simulink model "TST_InjCrv_PoI2AddCor"  (R2016b)
settings: Solver=FixedStepDiscrete  StartTime=0.0  StopTime=simTime  FixedStep=sampleTime  RelTol=1e-3
values from neighbouring files (symbols this model uses):
  testCase = 1    [initTST_InjCrv_PoI2AddCor_001.m]    (also in initTST_InjCrv_PoI2AddCor_002.m = 2; initTST_InjCrv_PoI2AddCor_003.m = 3; initTST_InjCrv_PoI2AddCor_004.m = 4)
libraries: simulink x29, UnitTest_Lib x24
(part 2 of 2)

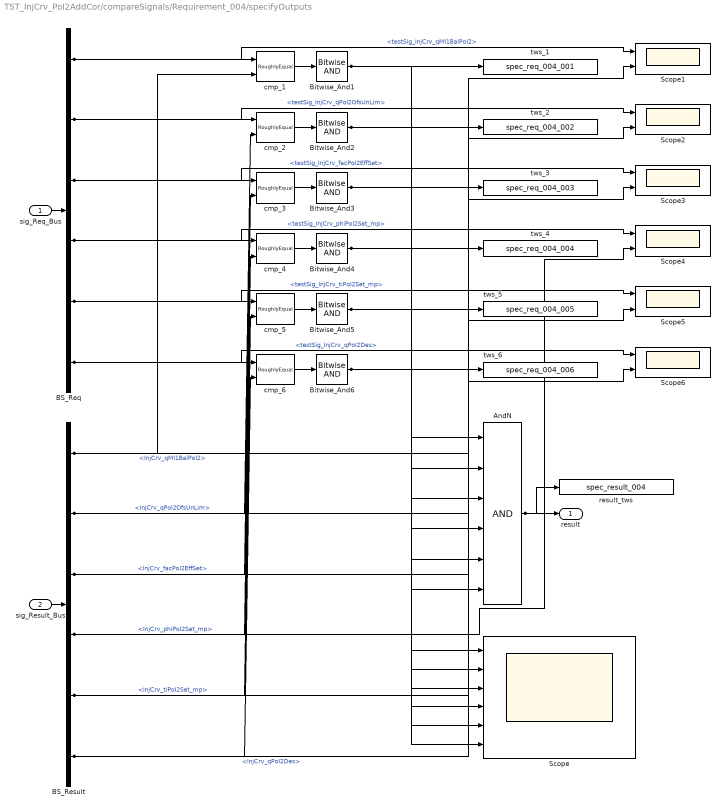
== system TST_InjCrv_PoI2AddCor/compareSignals/Requirement_004/specifyOutputs ==
  sig_Req_Bus : Inport
  sig_Result_Bus : Inport  Port=2
  AndN : Logic  Inputs=6
  BS_Req : BusSelector  OutputSignals=testSig_InjCrv_qMI1BalPoI2,testSig_InjCrv_qPoI2OfsUnLim,testSig_InjCrv_facPoI2EffSet,testSig_InjCrv_phiPoI2Set_mp,testSig_InjCrv_tiPoI2Set_mp,testSig_InjCrv_qPoI2Des
  BS_Result : BusSelector  OutputSignals=InjCrv_qMI1BalPoI2,InjCrv_qPoI2OfsUnLim,InjCrv_facPoI2EffSet,InjCrv_phiPoI2Set_mp,InjCrv_tiPoI2Set_mp,InjCrv_qPoI2Des
  Bitwise_And{1..6} (6 alike) : simulink/Logic and Bit Operations/Bitwise Operator  logicop=AND  UseBitMask=off  BitMask=bin2dec('11011001')  BitMaskRealWorld=Stored Integer
  Scope : Scope  NumInputPorts=6
  Scope{1..6} (6 alike) : Scope  NumInputPorts=2
  cmp_{1..6} (6 alike) : UnitTest_Lib/RoughlyEqual  slope=0.1
  result_tws : ToWorkspace  VariableName=spec_result_004
  tws_1 : ToWorkspace  VariableName=spec_req_004_001
  tws_2 : ToWorkspace  VariableName=spec_req_004_002
  tws_3 : ToWorkspace  VariableName=spec_req_004_003
  tws_4 : ToWorkspace  VariableName=spec_req_004_004
  tws_5 : ToWorkspace  VariableName=spec_req_004_005
  tws_6 : ToWorkspace  VariableName=spec_req_004_006
  result : Outport
  wires:
  sig_Req_Bus/1 -> BS_Req/1
  sig_Result_Bus/1 -> BS_Result/1
  AndN/1 -> result/1, result_tws/1
  BS_Req/1 -> cmp_1/1, Scope1/1  "<testSig_InjCrv_qMI1BalPoI2>"
  BS_Result/1 -> cmp_1/2, Scope1/2  "<InjCrv_qMI1BalPoI2>"
  cmp_1/1 -> Bitwise_And1/1
  Bitwise_And1/1 -> tws_1/1, AndN/1, Scope/1
  BS_Req/2 -> cmp_2/1, Scope2/1  "<testSig_InjCrv_qPoI2OfsUnLim>"
  BS_Result/2 -> cmp_2/2, Scope2/2  "<InjCrv_qPoI2OfsUnLim>"
  cmp_2/1 -> Bitwise_And2/1
  Bitwise_And2/1 -> tws_2/1, AndN/2, Scope/2
  BS_Req/3 -> cmp_3/1, Scope3/1  "<testSig_InjCrv_facPoI2EffSet>"
  BS_Result/3 -> cmp_3/2, Scope3/2  "<InjCrv_facPoI2EffSet>"
  cmp_3/1 -> Bitwise_And3/1
  Bitwise_And3/1 -> tws_3/1, AndN/3, Scope/3
  BS_Req/4 -> cmp_4/1, Scope4/1  "<testSig_InjCrv_phiPoI2Set_mp>"
  BS_Result/4 -> cmp_4/2, Scope4/2  "<InjCrv_phiPoI2Set_mp>"
  cmp_4/1 -> Bitwise_And4/1
  Bitwise_And4/1 -> tws_4/1, AndN/4, Scope/4
  BS_Req/5 -> cmp_5/1, Scope5/1  "<testSig_InjCrv_tiPoI2Set_mp>"
  BS_Result/5 -> cmp_5/2, Scope5/2  "<InjCrv_tiPoI2Set_mp>"
  cmp_5/1 -> Bitwise_And5/1
  Bitwise_And5/1 -> tws_5/1, AndN/5, Scope/5
  BS_Req/6 -> cmp_6/1, Scope6/1  "<testSig_InjCrv_qPoI2Des>"
  BS_Result/6 -> cmp_6/2, Scope6/2  "<InjCrv_qPoI2Des>"
  cmp_6/1 -> Bitwise_And6/1
  Bitwise_And6/1 -> tws_6/1, AndN/6, Scope/6
